simulink model "Stateflow2"  (R2025b)
settings: Solver=VariableStepAuto  StartTime=0.0  StopTime=10.0  RelTol=1e-3
settings Model: Creator=jujma  LastModifiedBy=jujma

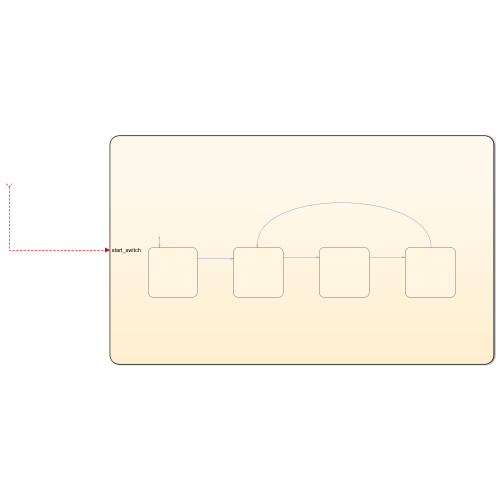
[thumbnail: Simulink's stored preview of the top-level diagram]
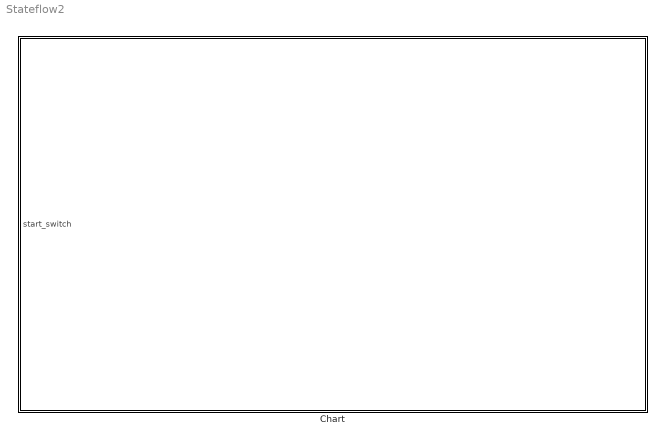
== system Stateflow2 ==
  Chart : Stateflow chart  TreatAsAtomicUnit=on
  wires:
  ? -> Chart/1(start_switch)

== stateflow chart Stateflow2/Chart ==
  state idle
    en:
    Start=0;
  state aiming
  state going
  state arrived
  arrived -> aiming
  (default) -> idle
  going -> arrived : reached
  aiming -> going : aligned
  idle -> aiming : [start_switch==1]
  data: start_switch input
